simulink model "telemetria_ahrs"  (R2020b)
settings: Solver=FixedStepAuto  StartTime=0.0  StopTime=inf  RelTol=1e-3  EnableMultiTasking=on
libraries: simulink_extras x11, svdutilitieslib x2, arduinolib x1
(part 1 of 2)
settings Model: SILPILModeSetting=veronly  ExtModeTrigDuration=2  Creator=ricca  LastModifiedBy=lapis-dspace
settings SolverCC: AutoInsertRateTranBlk=on
settings OptimizationCC: EnhancedBackFolding=on  PassReuseOutputArgsAs=Individual arguments  ZeroExternalMemoryAtStartup=off  ZeroInternalMemoryAtStartup=off  MaxStackSize=64  OptimizeBlockOrder=speed  DifferentSizesBufferReuse=on  OptimizationCustomize=off  EfficientTunableParamExpr=on
settings DebuggingCC: ParameterTunabilityLossMsg=error
settings HardwareCC: ProdBitPerPointer=32  ProdBitPerSizeT=32  ProdBitPerPtrDiffT=32  ProdLargestAtomicInteger=Long  ProdLargestAtomicFloat=Double  ProdWordSize=32  ProdHWDeviceType=ARM Compatible->ARM Cortex
settings SFSimCC: MATLABDynamicMemAlloc=off
settings RTWCC: Description=Embedded Coder  SystemTargetFile=ert.tlc  HardwareBoard=Arduino Due  TemplateMakefile=ert_default_tmf  Toolchain=Arduino ARM  BuildConfiguration=Faster Runs
settings CodeAppCC: ForceParamTrailComments=on  IgnoreCustomStorageClasses=off  OperatorAnnotations=on  SimulinkDataObjDesc=on  SFDataObjDesc=on  InsertBlockDesc=on
settings ERTTargetCC: SupportContinuousTime=on  SupportVariableSizeSignals=on  ExtModeTransport=3  ExtModeStaticAllocSize=24576  ExtModeMexFile=ext_xcp  ExtModeIntrfLevel=Level2 - Open

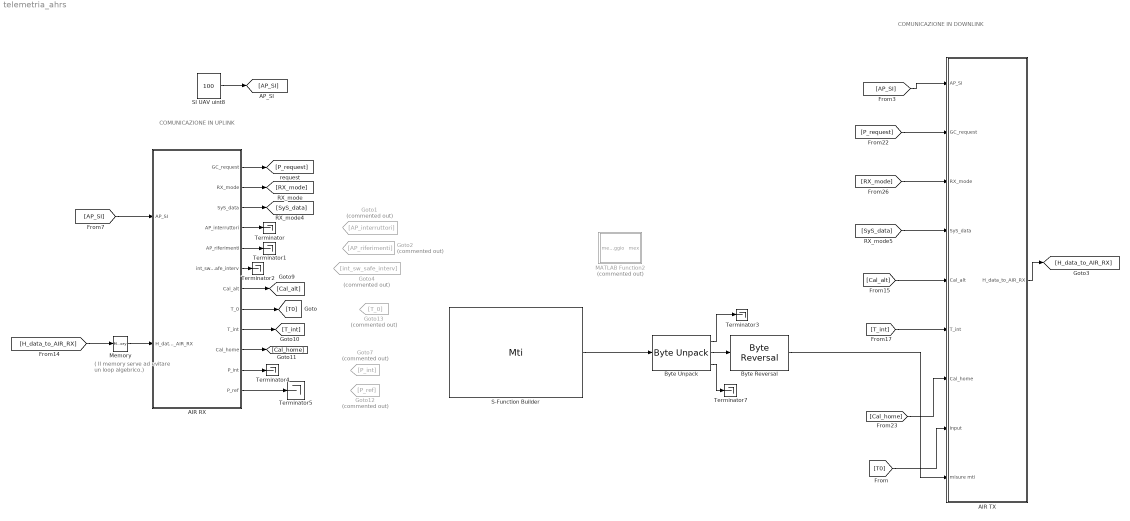
== system telemetria_ahrs ==
  note: ( Il memory serve ad evitare
      | un loop algebrico.)
  note: COMUNICAZIONE IN UPLINK
  note: COMUNICAZIONE IN DOWNLINK
  AIR RX : Subsystem
  AIR TX : Subsystem
  Byte Reversal : svdutilitieslib/Byte Reversal  numInp=1  blockPlatform=arduinoert
      settings: SourceProductBaseCode=ANDROID,ARDUINO,ML_ARDUINO,ECCORTEXA,ECCORTEXR,SC_BEAGLEBONE_BLUE,EC_FREEDOM_BOARD,EC_FRDM_K64F,INTEL_BLOCKSET,JETSONCPU,MICROBIT,NUCLEO,NVIDIA,PX4AUTOPILOTS,RASPPIIO,STMICRODIS,TIC2000,XILINX_BLOCKSET
  Byte Unpack : svdutilitieslib/Byte Unpack  dimensions={[4],[9],[1]}  datatypes={'uint8','single','uint8'}  byteAlign=1  blockPlatform=arduinoert
      settings: SourceProductBaseCode=ANDROID,ARDUINO,ML_ARDUINO,ECCORTEXA,ECCORTEXR,SC_BEAGLEBONE_BLUE,EC_FREEDOM_BOARD,EC_FRDM_K64F,INTEL_BLOCKSET,JETSONCPU,MICROBIT,NUCLEO,NVIDIA,PX4AUTOPILOTS,RASPPIIO,STMICRODIS,TIC2000,XILINX_BLOCKSET
  Goto1 : Goto  Commented=on  GotoTag=AP_interruttori
  Goto12 : Goto  Commented=on  GotoTag=P_ref
  Goto13 : Goto  Commented=on  GotoTag=T_0
  Goto2 : Goto  Commented=on  GotoTag=AP_riferimenti
  Goto4 : Goto  Commented=on  GotoTag=int_sw_safe_interv
  Goto7 : Goto  Commented=on  GotoTag=P_int
  MATLAB Function2 : MATLAB Function  Commented=on  TreatAsAtomicUnit=on
  Memory : Memory
  S-Function Builder : S-Function  InitFcn=try, set_param(gcb,'FunctionName','Mti'), end  FunctionName=Mti  SFunctionModules=Mti_wrapper  SFunctionDeploymentMode=off  EnableBusSupport=off  mask(S-Function Builder){}
      mask help: Simulink:masks:SFunctionBuilder_MD
      mask init:
      | val = [[.9  0.75 0.75 1 1 .9 .9 1]',[1 1 0.75 0.75 .9 .9 1 .9]'];try , sys = get_param(gcb,'SfunBuilderFcnName');if isempty(sys), sys = get_param(gcb,'FunctionName'); end,catch, sys = get_param(gcb,'FunctionName'); end
      settings: CopyFcn=set_param(gcbh,'LinkStatus','none')  PreSaveFcn=try, set_param(gcb,'FunctionName','Mti'), end  OpenFcn=sfunctionwizard(gcbh)
      mask Display: plot(val(:,1),val(:,2)),disp(sys),port_label('output',1,'messaggio')
  SI UAV uint8 : Constant  Value=100  OutDataTypeStr=uint8
  Terminator{,1..5,7} (7 alike) : Terminator
  wires:
  AIR RX/7(Cal_alt) -> [Cal_alt]
  AIR RX/12(P_ref) -> Terminator5/1
  [AP_SI] -> AIR RX/1(AP_SI)
  [H_data_to_AIR_RX] -> Memory/1
  AIR RX/8(T_0) -> [T0]
  AIR RX/10(Cal_home) -> [Cal_home]
  AIR RX/9(T_int) -> [T_int]
  AIR RX/6(int_sw_safe_interv) -> Terminator2/1
  AIR RX/1(GC_request) -> [P_request]
  Memory/1 -> AIR RX/2(H_data_to_AIR_RX)
  AIR RX/2(RX_mode) -> [RX_mode]
  AIR RX/5(AP_riferimenti) -> Terminator1/1
  AIR RX/11(P_int) -> Terminator4/1
  AIR RX/4(AP_interruttori) -> Terminator/1
  AIR RX/3(SyS_data) -> [SyS_data]
  SI UAV uint8/1 -> [AP_SI]
  AIR TX/1(H_data_to_AIR_RX) -> [H_data_to_AIR_RX]
  [AP_SI] -> AIR TX/1(AP_SI)
  [Cal_alt] -> AIR TX/5(Cal_alt)
  [P_request] -> AIR TX/2(GC_request)
  [T_int] -> AIR TX/6(T_int)
  [RX_mode] -> AIR TX/3(RX_mode)
  [SyS_data] -> AIR TX/4(SyS_data)
  [Cal_home] -> AIR TX/7(Cal_home)
  [T0] -> AIR TX/8(Input)
  Byte Unpack/1 -> Terminator3/1
  Byte Unpack/2 -> Byte Reversal/1
  Byte Unpack/3 -> Terminator7/1
  S-Function Builder/1 -> Byte Unpack/1
  Byte Reversal/1 -> AIR TX/9(misure mti)

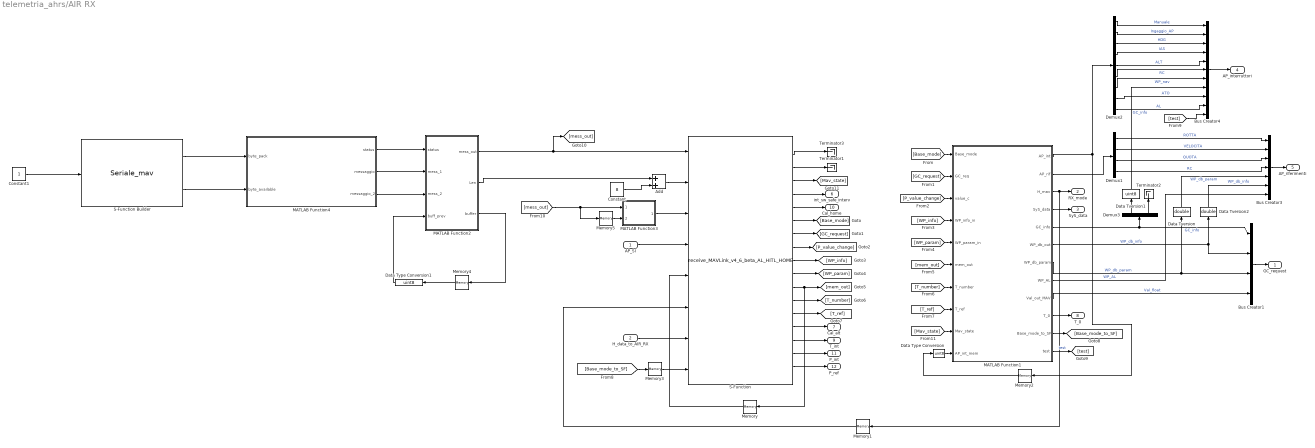
== system telemetria_ahrs/AIR RX ==
  AP_SI : Inport
  H_data_to_AIR_RX : Inport  Port=2
  Add : Sum  AccumDataTypeStr=int32
  Bus Creator1 : BusCreator  Inputs=4
  Bus Creator3 : BusCreator  Inputs=7
  Bus Creator4 : BusCreator  Inputs=11
  Constant : Constant  Value=8  OutDataTypeStr=int32  SampleTime=-1
  Constant1 : Constant  OutDataTypeStr=uint8
  Data Tversion : DataTypeConversion  OutDataTypeStr=double
  Data Tversion1 : DataTypeConversion  OutDataTypeStr=uint8
  Data Tversion2 : DataTypeConversion  OutDataTypeStr=double
  Data Type Conversion : DataTypeConversion  OutDataTypeStr=uint8
  Data Type Conversion1 : DataTypeConversion  OutDataTypeStr=uint8
  Demux1 : Demux
  Demux2 : Demux  Outputs=9
  Demux3 : Demux  Outputs=[1 2]
  MATLAB Function1 : MATLAB Function  TreatAsAtomicUnit=on
  MATLAB Function2 : MATLAB Function  TreatAsAtomicUnit=on
  MATLAB Function3 : MATLAB Function  TreatAsAtomicUnit=on
  MATLAB Function4 : MATLAB Function  TreatAsAtomicUnit=on
  Memory : Memory  InheritSampleTime=on
  Memory1 : Memory  InheritSampleTime=on
  Memory2 : Memory  InitialCondition=[0 0 0 0 0 0 0 0 0]
  Memory3 : Memory
  Memory4 : Memory  InitialCondition=uint8(zeros(3,100))  InheritSampleTime=on
  Memory5 : Memory  InheritSampleTime=on
  S-Function : S-Function  FunctionName=receive_MAVLink_v4_6_beta_AL_HITL_HOME  SFunctionModules='receive_MAVLink_v4_6_beta_AL_HITL_HOME_wrapper'  SFunctionDeploymentMode=off  EnableBusSupport=off
  S-Function Builder : S-Function  InitFcn=try, set_param(gcb,'FunctionName','Seriale_mav'), end  FunctionName=Seriale_mav  SFunctionModules=Seriale_mav_wrapper  SFunctionDeploymentMode=off  EnableBusSupport=off  mask(S-Function Builder){}
      mask help: Simulink:masks:SFunctionBuilder_MD
      mask init: same as telemetria_ahrs/S-Function Builder
      settings: CopyFcn=set_param(gcbh,'LinkStatus','none')  PreSaveFcn=try, set_param(gcb,'FunctionName','Seriale_mav'), end  OpenFcn=sfunctionwizard(gcbh)
      mask Display: plot(val(:,1),val(:,2)),disp(sys),port_label('input',1,'inutile'),port_label('output',1,'Messaggio'),port_label('output',2,'serial_available')
  Terminator1 : Terminator
  Terminator2 : Terminator
  Terminator3 : Terminator
  GC_request : Outport  VectorParamsAs1DForOutWhenUnconnected=off
  RX_mode : Outport  Port=2  VectorParamsAs1DForOutWhenUnconnected=off
  SyS_data : Outport  Port=3  VectorParamsAs1DForOutWhenUnconnected=off
  AP_interruttori : Outport  Port=4  VectorParamsAs1DForOutWhenUnconnected=off
  AP_riferimenti : Outport  Port=5  VectorParamsAs1DForOutWhenUnconnected=off
  int_sw_safe_interv : Outport  Port=6  VectorParamsAs1DForOutWhenUnconnected=off
  Cal_alt : Outport  Port=7  VectorParamsAs1DForOutWhenUnconnected=off
  T_0 : Outport  Port=8  VectorParamsAs1DForOutWhenUnconnected=off
  T_int : Outport  Port=9  VectorParamsAs1DForOutWhenUnconnected=off
  Cal_home : Outport  Port=10  VectorParamsAs1DForOutWhenUnconnected=off
  P_int : Outport  Port=11  VectorParamsAs1DForOutWhenUnconnected=off
  P_ref : Outport  Port=12  VectorParamsAs1DForOutWhenUnconnected=off
  wires:
  H_data_to_AIR_RX/1 -> S-Function/7
  Memory1/1 -> S-Function/6
  Memory/1 -> S-Function/5
  Memory3/1 -> S-Function/8
  AP_SI/1 -> S-Function/4
  S-Function/5 -> Cal_home/1
  S-Function/4 -> int_sw_safe_interv/1
  S-Function/3 -> [Mav_state]
  S-Function/2 -> Terminator1/1
  S-Function/1 -> Terminator3/1
  S-Function/15 -> T_int/1
  S-Function/14 -> Cal_alt/1
  S-Function/13 -> [T_ref]
  S-Function/12 -> [T_number]
  S-Function/11 -> Memory/1, [mem_out]
  S-Function/10 -> [WP_param]
  S-Function/9 -> [WP_info]
  S-Function/8 -> [P_value_change]
  S-Function/6 -> [Base_mode]
  S-Function/7 -> [GC_request]
  Demux2/6 -> Bus Creator4/6  "RC"
  Data Tversion1/1 -> Bus Creator4/8  "GC_info"
  Memory2/1 -> Data Type Conversion/1
  Bus Creator1/1 -> GC_request/1
  Demux1/2 -> Bus Creator3/2  "VELOCITA"
  Demux2/5 -> Bus Creator4/5  "ALT"
  Demux2/1 -> Bus Creator4/1  "Manuale"
  Demux2/3 -> Bus Creator4/3  "HDG"
  [P_value_change] -> MATLAB Function1/3(value_c)
  Demux1/4 -> Bus Creator3/4  "RC"
  MATLAB Function1/2(AP_rif) -> Demux1/1
  Demux2/8 -> Bus Creator4/9  "ATO"
  MATLAB Function1/7(WP_db_param) -> Bus Creator1/3, Data Tversion/1  "WP_db_param"
  [GC_request] -> MATLAB Function1/2(GC_req)
  Demux2/2 -> Bus Creator4/2  "Ingaggio_AP"
  [mem_out] -> MATLAB Function1/6(mem_out)
  Bus Creator4/1 -> AP_interruttori/1
  MATLAB Function1/4(SyS_data) -> SyS_data/1
  MATLAB Function1/6(WP_db_out) -> Data Tversion2/1, Bus Creator1/2  "WP_db_info"
  [Mav_state] -> MATLAB Function1/9(Mav_state)
  Demux2/7 -> Bus Creator4/7  "WP_nav"
  [T_ref] -> MATLAB Function1/8(T_ref)
  Data Type Conversion/1 -> MATLAB Function1/10(AP_int_mem)
  Data Tversion2/1 -> Bus Creator3/6  "WP_db_info"
  Demux3/2 -> Terminator2/1
  [Base_mode] -> MATLAB Function1/1(Base_mode)
  [WP_param] -> MATLAB Function1/5(WP_param_in)
  Data Tversion/1 -> Bus Creator3/5  "WP_db_param"
  Demux3/1 -> Data Tversion1/1
  MATLAB Function1/3(H_mav) -> Memory1/1, RX_mode/1
  MATLAB Function1/9(Val_out_MAV) -> Bus Creator1/4  "Val_float"
  Bus Creator3/1 -> AP_riferimenti/1
  [T_number] -> MATLAB Function1/7(T_number)
  MATLAB Function1/5(GC_info) -> Demux3/1, Bus Creator1/1  "GC_info"
  MATLAB Function1/1(AP_int) -> Demux2/1, Memory2/1
  [WP_info] -> MATLAB Function1/4(WP_info_in)
  [Base_mode_to_SF] -> Memory3/1
  MATLAB Function1/11(Base_mode_to_SF) -> [Base_mode_to_SF]
  Demux1/3 -> Bus Creator3/3  "QUOTA"
  MATLAB Function1/12(test) -> [test]  "test"
  Demux2/4 -> Bus Creator4/4  "IAS"
  [test] -> Bus Creator4/11
  Demux1/1 -> Bus Creator3/1  "ROTTA"
  MATLAB Function1/8(WP_AL) -> Bus Creator3/7  "WP_AL"
  MATLAB Function1/10(T_0) -> T_0/1
  Demux2/9 -> Bus Creator4/10  "AL"
  MATLAB Function4/3(messaggio_2) -> MATLAB Function2/3(mess_2)
  MATLAB Function2/2(Len) -> Add/1
  MATLAB Function4/1(status) -> MATLAB Function2/1(status)
  MATLAB Function4/2(messaggio) -> MATLAB Function2/2(mess_1)
  Memory4/1 -> Data Type Conversion1/1
  MATLAB Function2/3(buffer) -> Memory4/1
  Constant/1 -> Add/2
  MATLAB Function2/1(mess_out) -> S-Function/1, [mess_out]
  MATLAB Function3/1(new_mex) -> S-Function/3
  Add/1 -> S-Function/2
  Data Type Conversion1/1 -> MATLAB Function2/4(buff_prev)
  Memory5/1 -> MATLAB Function3/2(mess_out_prev)
  [mess_out] -> Memory5/1, MATLAB Function3/1(mess_out)
  S-Function Builder/2 -> MATLAB Function4/2(byte_available)
  S-Function Builder/1 -> MATLAB Function4/1(byte_pack)
  Constant1/1 -> S-Function Builder/1
  S-Function/16 -> P_int/1
  S-Function/17 -> P_ref/1

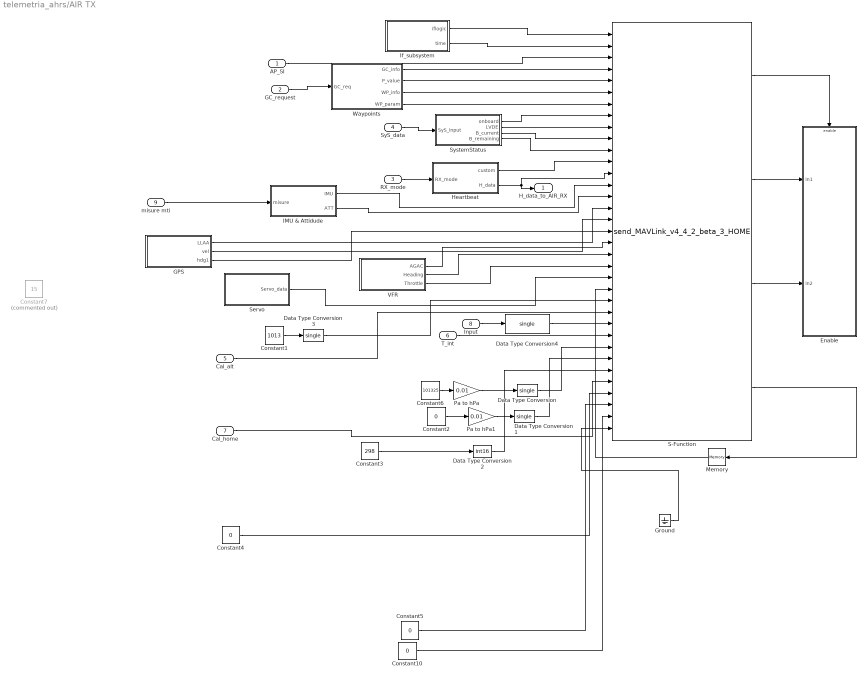
== system telemetria_ahrs/AIR TX ==
  AP_SI : Inport
  GC_request : Inport  Port=2
  RX_mode : Inport  Port=3
  SyS_data : Inport  Port=4
  Cal_alt : Inport  Port=5
  T_int : Inport  Port=6
  Cal_home : Inport  Port=7
  Input : Inport  Port=8
  misure mti : Inport  Port=9
  Constant1 : Constant  Value=1013
  Constant{2,4..5,10} (4 alike) : Constant  Value=0
  Constant3 : Constant  Value=298
  Constant6 : Constant  Value=101325
  Constant7 : Constant  Commented=on  Value=15
  Data Type Conversion{,1,3..4} (4 alike) : DataTypeConversion  OutDataTypeStr=single
  Data Type Conversion2 : DataTypeConversion  OutDataTypeStr=int16
  "Enable " : Subsystem  TreatAsAtomicUnit=on
  GPS : Subsystem  SystemSampleTime=0.02
  Ground : Ground
  Heartbeat : Subsystem  SystemSampleTime=1
  IMU & Attidude : Subsystem  SystemSampleTime=0.04
  If_subsystem : Subsystem
  Memory : Memory
  Pa to hPa : Gain  Gain=0.01
  Pa to hPa1 : Gain  Gain=0.01
  S-Function : S-Function  FunctionName=send_MAVLink_v4_4_2_beta_3_HOME  SFunctionModules='send_MAVLink_v4_4_2_beta_3_HOME_wrapper'  SFunctionDeploymentMode=off  EnableBusSupport=off
  Servo : Subsystem  SystemSampleTime=0.5
  SystemStatus : Subsystem  SystemSampleTime=0.2
  VFR : Subsystem  SystemSampleTime=0.5
  Waypoints : Subsystem  SystemSampleTime=1
  H_data_to_AIR_RX : Outport  VectorParamsAs1DForOutWhenUnconnected=off
  wires:
  If_subsystem/2(time) -> S-Function/2
  If_subsystem/1(iflogic) -> S-Function/1
  VFR/2(Heading) -> S-Function/20
  Heartbeat/2(H_data) -> H_data_to_AIR_RX/1, S-Function/13
  RX_mode/1 -> Heartbeat/1(RX_mode)
  S-Function/1 -> "Enable "/Enable
  Input/1 -> Data Type Conversion4/1
  AP_SI/1 -> S-Function/3
  Constant2/1 -> Pa to hPa1/1
  SyS_data/1 -> SystemStatus/1(SyS_input)
  S-Function/3 -> "Enable "/2(In2)
  SystemStatus/1(onboard) -> S-Function/8
  SystemStatus/4(B_remaining) -> S-Function/11
  T_int/1 -> S-Function/27
  SystemStatus/2(LVDE) -> S-Function/9
  Heartbeat/1(custom) -> S-Function/12
  Cal_alt/1 -> S-Function/25
  GC_request/1 -> Waypoints/1(GC_req)
  S-Function/4 -> Memory/1
  S-Function/2 -> "Enable "/1(In1)
  GPS/3(hdg1) -> S-Function/18
  Waypoints/2(P_value) -> S-Function/5
  IMU & Attidude/2(ATT) -> S-Function/15
  Memory/1 -> S-Function/23
  Data Type Conversion1/1 -> S-Function/29
  Waypoints/1(GC_info) -> S-Function/4
  Servo/1(Servo_data) -> S-Function/22
  GPS/2(vel) -> S-Function/17
  IMU & Attidude/1(IMU) -> S-Function/14
  Constant3/1 -> Data Type Conversion2/1
  Waypoints/3(WP_info) -> S-Function/6
  Pa to hPa1/1 -> Data Type Conversion1/1
  Data Type Conversion3/1 -> S-Function/24
  GPS/1(LLAA) -> S-Function/16
  Data Type Conversion2/1 -> S-Function/30
  Constant10/1 -> S-Function/34
  SystemStatus/3(B_current) -> S-Function/10
  Cal_home/1 -> S-Function/31
  VFR/3(Throttle) -> S-Function/21
  Waypoints/4(WP_param) -> S-Function/7
  Constant4/1 -> S-Function/32
  VFR/1(AGAC) -> S-Function/19
  Constant5/1 -> S-Function/33
  Ground/1 -> S-Function/35
  Constant1/1 -> Data Type Conversion3/1
  Constant6/1 -> Pa to hPa/1
  Data Type Conversion/1 -> S-Function/28
  Pa to hPa/1 -> Data Type Conversion/1
  Data Type Conversion4/1 -> S-Function/26
  misure mti/1 -> IMU & Attidude/1(misure)

== system telemetria_ahrs/AIR TX/Enable  ==
  In1 : Inport
  In2 : Inport  Port=2
  Enable : EnablePort
  Chart : Stateflow chart  TreatAsAtomicUnit=on
  wires:
  In2/1 -> Chart/2(Len)
  In1/1 -> Chart/1(datain)

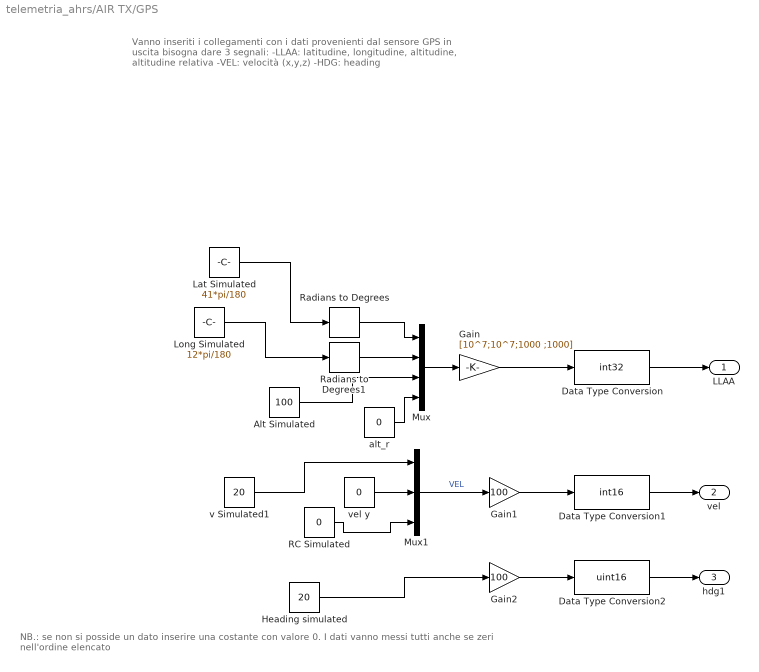
== system telemetria_ahrs/AIR TX/GPS ==
  note: NB.: se non si posside un dato inserire una costante con valore 0. I dati vanno messi tutti anche se zeri nell'ordine elencato
  note: Vanno inseriti i collegamenti con i dati provenienti dal sensore GPS
      | in uscita bisogna dare 3 segnali:
      |
      | -LLAA: latitudine, longitudine, altitudine, altitudine relativa
      | -VEL: velocità (x,y,z)
      | -HDG: heading
  Alt Simulated : Constant  Value=100
  Data Type Conversion : DataTypeConversion  OutDataTypeStr=int32  RndMeth=Simplest
  Data Type Conversion1 : DataTypeConversion  OutDataTypeStr=int16  RndMeth=Simplest
  Data Type Conversion2 : DataTypeConversion  OutDataTypeStr=uint16  RndMeth=Simplest
  Gain : Gain  Gain=[10^7;10^7;1000 ;1000]
  Gain1 : Gain  Gain=100
  Gain2 : Gain  Gain=100
  Heading simulated : Constant  Value=20
  Lat Simulated : Constant  Value=41*pi/180
  Long Simulated : Constant  Value=12*pi/180
  Mux : Mux
  Mux1 : Mux  Inputs=3
  RC Simulated : Constant  Value=0
  Radians to Degrees : simulink_extras/Transformations/Radians to Degrees
  Radians to Degrees1 : simulink_extras/Transformations/Radians to Degrees
  alt_r : Constant  Value=0
  v Simulated1 : Constant  Value=20
  vel y : Constant  Value=0  OutDataTypeStr=double
  LLAA : Outport  VectorParamsAs1DForOutWhenUnconnected=off
  vel : Outport  Port=2  VectorParamsAs1DForOutWhenUnconnected=off
  hdg1 : Outport  Port=3  VectorParamsAs1DForOutWhenUnconnected=off
  wires:
  Lat Simulated/1 -> Radians to Degrees/1
  Long Simulated/1 -> Radians to Degrees1/1
  Alt Simulated/1 -> Mux/3
  Gain2/1 -> Data Type Conversion2/1
  Data Type Conversion/1 -> LLAA/1
  Gain/1 -> Data Type Conversion/1
  Data Type Conversion1/1 -> vel/1
  Radians to Degrees1/1 -> Mux/2
  Radians to Degrees/1 -> Mux/1
  RC Simulated/1 -> Mux1/3
  vel y/1 -> Mux1/2
  Heading simulated/1 -> Gain2/1
  Mux/1 -> Gain/1
  v Simulated1/1 -> Mux1/1
  Mux1/1 -> Gain1/1  "VEL"
  Data Type Conversion2/1 -> hdg1/1
  alt_r/1 -> Mux/4
  Gain1/1 -> Data Type Conversion1/1

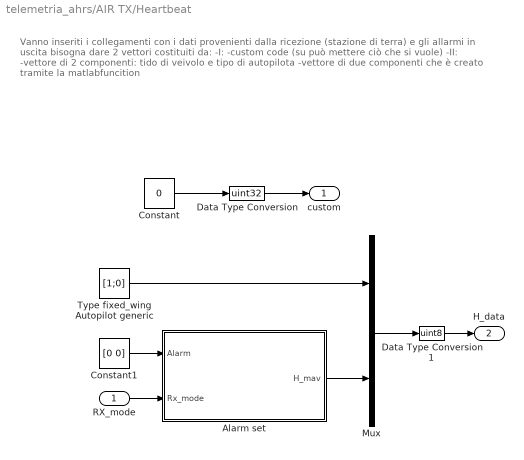
== system telemetria_ahrs/AIR TX/Heartbeat ==
  note: Vanno inseriti i collegamenti con i dati provenienti dalla ricezione (stazione di terra) e gli allarmi
      | in uscita bisogna dare 2 vettori costituiti da:
      | -I:
      | -custom code (su può mettere ciò che si vuole)
      | -II:
      | -vettore di 2 componenti: tido di veivolo e tipo di autopilota
      | -vettore di due componenti che è creato tramite la matlabfuncition
  RX_mode : Inport
  Alarm set : MATLAB Function  TreatAsAtomicUnit=on
  Constant : Constant  Value=0
  Constant1 : Constant  Value=[0 0]
  Data Type Conversion : DataTypeConversion  OutDataTypeStr=uint32
  Data Type Conversion1 : DataTypeConversion  OutDataTypeStr=uint8
  Mux : Mux  Inputs=2
  Type fixed_wing Autopilot generic : Constant  Value=[1;0]  OutDataTypeStr=uint8
  custom : Outport  VectorParamsAs1DForOutWhenUnconnected=off
  H_data : Outport  Port=2  VectorParamsAs1DForOutWhenUnconnected=off
  wires:
  Constant/1 -> Data Type Conversion/1
  Data Type Conversion1/1 -> H_data/1
  Data Type Conversion/1 -> custom/1
  RX_mode/1 -> Alarm set/2(Rx_mode)
  Constant1/1 -> Alarm set/1(Alarm)
  Type fixed_wing Autopilot generic/1 -> Mux/1
  Alarm set/1(H_mav) -> Mux/2
  Mux/1 -> Data Type Conversion1/1

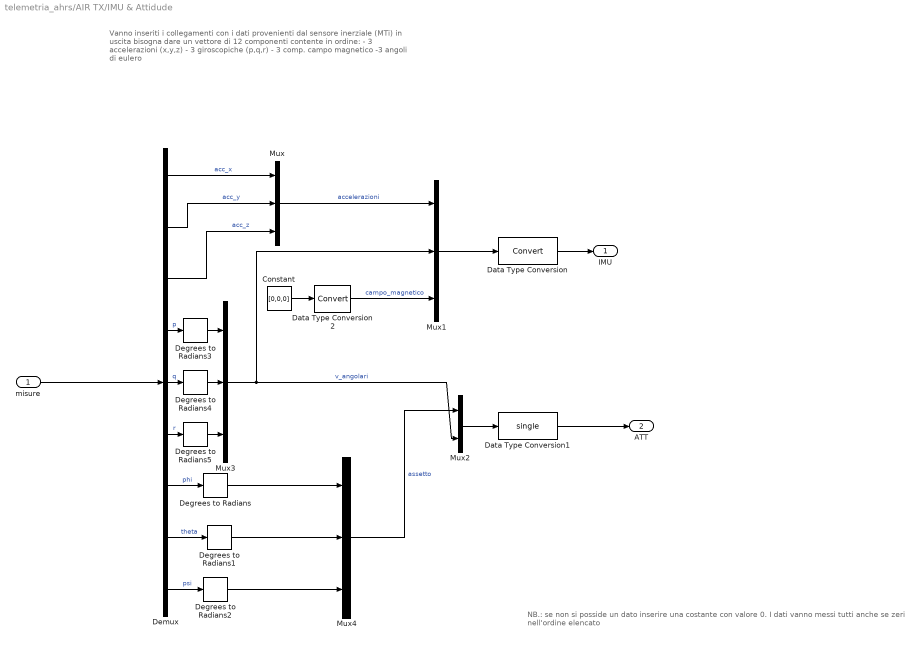
== system telemetria_ahrs/AIR TX/IMU & Attidude ==
  note: Vanno inseriti i collegamenti con i dati provenienti dal sensore inerziale (MTi)
      | in uscita bisogna dare un vettore di 12 componenti contente in ordine:
      | - 3 accelerazioni (x,y,z)
      | - 3 giroscopiche (p,q,r)
      | - 3 comp. campo magnetico
      | -3 angoli di eulero
  note: NB.: se non si posside un dato inserire una costante con valore 0. I dati vanno messi tutti anche se zeri nell'ordine elencato
  misure : Inport
  Constant : Constant  Value=[0,0,0]
  Data Type Conversion : DataTypeConversion
  Data Type Conversion1 : DataTypeConversion  OutDataTypeStr=single
  Data Type Conversion2 : DataTypeConversion
  Degrees to Radians{,1..5} (6 alike) : simulink_extras/Transformations/Degrees to Radians
  Demux : Demux  Outputs=9
  Mux{,1,3..4} (4 alike) : Mux  Inputs=3
  Mux2 : Mux  Inputs=2
  IMU : Outport  VectorParamsAs1DForOutWhenUnconnected=off
  ATT : Outport  Port=2  VectorParamsAs1DForOutWhenUnconnected=off
  wires:
  Demux/4 -> Degrees to Radians3/1  "p"
  Demux/6 -> Degrees to Radians5/1  "r"
  Demux/7 -> Degrees to Radians/1  "phi"
  Demux/9 -> Degrees to Radians2/1  "psi"
  Demux/5 -> Degrees to Radians4/1  "q"
  Demux/8 -> Degrees to Radians1/1  "theta"
  misure/1 -> Demux/1
  Mux/1 -> Mux1/1  "accelerazioni"
  Demux/3 -> Mux/3  "acc_z"
  Mux4/1 -> Mux2/1  "assetto"
  Demux/2 -> Mux/2  "acc_y"
  Mux3/1 -> Mux1/2, Mux2/2  "v_angolari"
  Demux/1 -> Mux/1  "acc_x"
  Mux1/1 -> Data Type Conversion/1
  Mux2/1 -> Data Type Conversion1/1
  Data Type Conversion1/1 -> ATT/1
  Data Type Conversion/1 -> IMU/1
  Constant/1 -> Data Type Conversion2/1
  Data Type Conversion2/1 -> Mux1/3  "campo_magnetico"
  Degrees to Radians2/1 -> Mux4/3
  Degrees to Radians3/1 -> Mux3/1
  Degrees to Radians4/1 -> Mux3/2
  Degrees to Radians5/1 -> Mux3/3
  Degrees to Radians/1 -> Mux4/1
  Degrees to Radians1/1 -> Mux4/2

== system telemetria_ahrs/AIR TX/If_subsystem ==
  note: Blocco per la temporizzazione dell'invio dei messaggi
  Data Type Conversion3 : DataTypeConversion  OutDataTypeStr=uint32  RndMeth=Simplest
  Gain : Gain  Gain=100
  Subsystem : Subsystem
  iflogic_function : MATLAB Function  TreatAsAtomicUnit=on
  iflogic : Outport  VectorParamsAs1DForOutWhenUnconnected=off
  time : Outport  Port=2  VectorParamsAs1DForOutWhenUnconnected=off
  wires:
  Subsystem/3(time) -> Gain/1
  Subsystem/2(H_10) -> iflogic_function/2(H10)
  Subsystem/1(H_50) -> iflogic_function/1(H50)
  Gain/1 -> Data Type Conversion3/1
  Data Type Conversion3/1 -> time/1
  iflogic_function/1(iflogic) -> iflogic/1

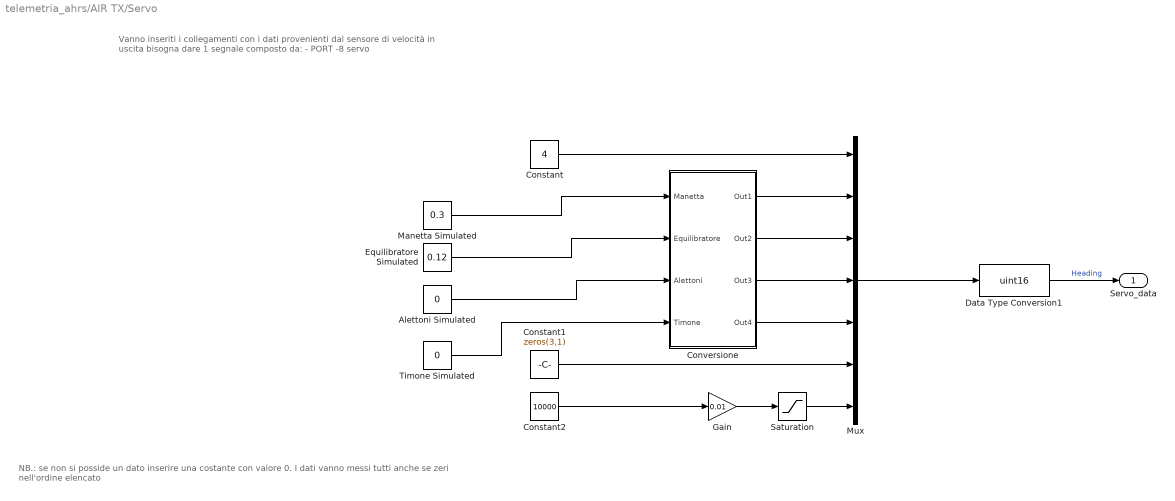
== system telemetria_ahrs/AIR TX/Servo ==
  note: NB.: se non si posside un dato inserire una costante con valore 0. I dati vanno messi tutti anche se zeri nell'ordine elencato
  note: Vanno inseriti i collegamenti con i dati provenienti dal sensore di velocità
      | in uscita bisogna dare 1 segnale composto da:
      |
      | -  PORT
      | -8 servo
  Alettoni Simulated : Constant  Value=0
  Constant : Constant  Value=4
  Constant1 : Constant  Value=zeros(3,1)
  Constant2 : Constant  Value=10000
  Conversione : Subsystem
  Data Type Conversion1 : DataTypeConversion  OutDataTypeStr=uint16  RndMeth=Simplest
  Equilibratore Simulated : Constant  Value=0.12
  Gain : Gain  Gain=0.01
  Manetta Simulated : Constant  Value=0.3
  Mux : Mux  Inputs=7
  Saturation : Saturate  UpperLimit=4000  LowerLimit=0
  Timone Simulated : Constant  Value=0
  Servo_data : Outport  VectorParamsAs1DForOutWhenUnconnected=off
  wires:
  Constant2/1 -> Gain/1
  Equilibratore Simulated/1 -> Conversione/2(Equilibratore)
  Alettoni Simulated/1 -> Conversione/3(Alettoni)
  Timone Simulated/1 -> Conversione/4(Timone)
  Manetta Simulated/1 -> Conversione/1(Manetta)
  Conversione/3(Out3) -> Mux/4
  Constant1/1 -> Mux/6
  Conversione/1(Out1) -> Mux/2
  Mux/1 -> Data Type Conversion1/1
  Constant/1 -> Mux/1
  Data Type Conversion1/1 -> Servo_data/1  "Heading"
  Conversione/4(Out4) -> Mux/5
  Saturation/1 -> Mux/7
  Gain/1 -> Saturation/1
  Conversione/2(Out2) -> Mux/3

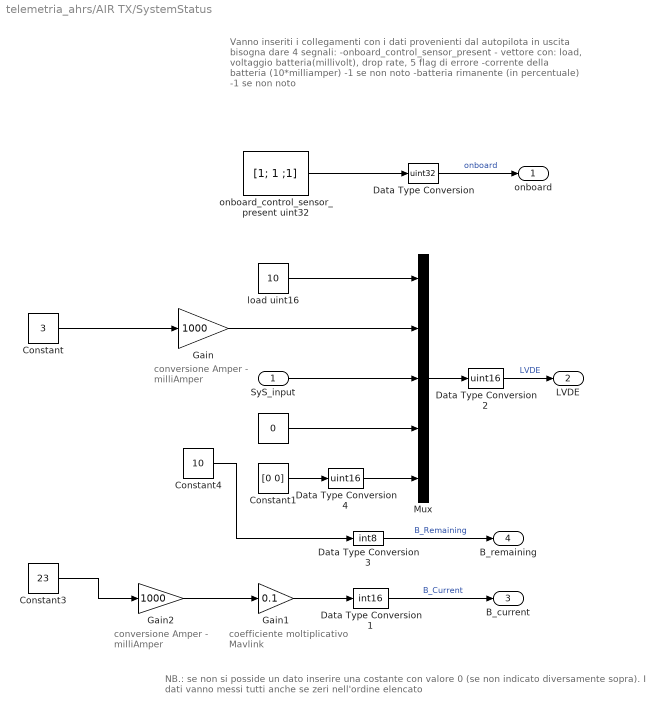
== system telemetria_ahrs/AIR TX/SystemStatus ==
  note: coefficiente moltiplicativo Mavlink
  note: conversione
      | Amper - milliAmper
  note: NB.: se non si posside un dato inserire una costante con valore 0 (se non indicato diversamente sopra).
      | I dati vanno messi tutti anche se zeri nell'ordine elencato
  note: Vanno inseriti i collegamenti con i dati provenienti dal autopilota
      | in uscita bisogna dare 4 segnali:
      |
      | -onboard_control_sensor_present
      | - vettore con: load, voltaggio batteria(millivolt), drop rate, 5 flag di errore
      | -corrente della batteria (10*milliamper) -1 se non noto
      | -batteria rimanente (in percentuale) -1 se non noto
  note: conversione
      | Amper - milliAmper
  SyS_input : Inport
  " " : Constant  Value=0  OutDataTypeStr=uint16
  Constant : Constant  Value=3
  Constant1 : Constant  Value=[0 0]
  Constant3 : Constant  Value=23
  Constant4 : Constant  Value=10
  Data Type Conversion : DataTypeConversion  OutDataTypeStr=uint32
  Data Type Conversion1 : DataTypeConversion  OutDataTypeStr=int16
  Data Type Conversion2 : DataTypeConversion  OutDataTypeStr=uint16
  Data Type Conversion3 : DataTypeConversion  OutDataTypeStr=int8
  Data Type Conversion4 : DataTypeConversion  OutDataTypeStr=uint16
  Gain : Gain  Gain=1000  OutDataTypeStr=uint16
  Gain1 : Gain  Gain=0.1  OutDataTypeStr=int16
  Gain2 : Gain  Gain=1000  OutDataTypeStr=int16
  Mux : Mux  Inputs=5
  load uint16 : Constant  Value=10  OutDataTypeStr=uint16
  onboard_control_sensor_present uint32 : Constant  Value=[1; 1 ;1]  OutDataTypeStr=uint32
  onboard : Outport  VectorParamsAs1DForOutWhenUnconnected=off
  LVDE : Outport  Port=2  VectorParamsAs1DForOutWhenUnconnected=off
  B_current : Outport  Port=3  VectorParamsAs1DForOutWhenUnconnected=off
  B_remaining : Outport  Port=4  VectorParamsAs1DForOutWhenUnconnected=off
  wires:
  Gain2/1 -> Gain1/1
  Gain1/1 -> Data Type Conversion1/1
  " "/1 -> Mux/4
  Data Type Conversion4/1 -> Mux/5
  Constant1/1 -> Data Type Conversion4/1
  SyS_input/1 -> Mux/3
  Data Type Conversion3/1 -> B_remaining/1  "B_Remaining"
  Data Type Conversion1/1 -> B_current/1  "B_Current"
  Data Type Conversion2/1 -> LVDE/1  "LVDE"
  Data Type Conversion/1 -> onboard/1  "onboard"
  Mux/1 -> Data Type Conversion2/1
  Gain/1 -> Mux/2
  load uint16/1 -> Mux/1
  onboard_control_sensor_present uint32/1 -> Data Type Conversion/1
  Constant/1 -> Gain/1
  Constant4/1 -> Data Type Conversion3/1
  Constant3/1 -> Gain2/1

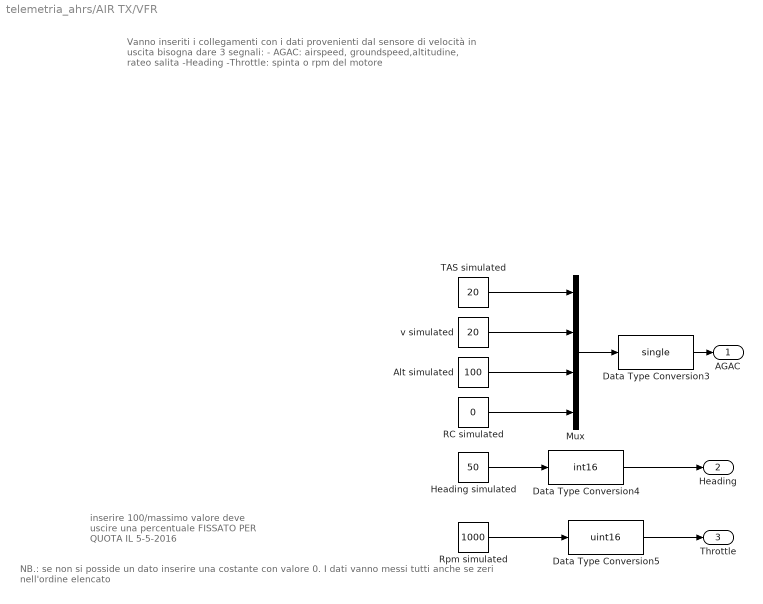
== system telemetria_ahrs/AIR TX/VFR ==
  note: NB.: se non si posside un dato inserire una costante con valore 0. I dati vanno messi tutti anche se zeri nell'ordine elencato
  note: Vanno inseriti i collegamenti con i dati provenienti dal sensore di velocità
      | in uscita bisogna dare 3 segnali:
      |
      | -  AGAC: airspeed, groundspeed,altitudine, rateo salita
      | -Heading
      | -Throttle: spinta o rpm del motore
  note: inserire 100/massimo valore
      | deve uscire una percentuale
      | FISSATO PER QUOTA IL 5-5-2016
  " Heading simulated" : Constant  Value=50
  Alt simulated : Constant  Value=100
  Data Type Conversion3 : DataTypeConversion  OutDataTypeStr=single
  Data Type Conversion4 : DataTypeConversion  OutDataTypeStr=int16
  Data Type Conversion5 : DataTypeConversion  OutDataTypeStr=uint16
  Mux : Mux
  RC simulated : Constant  Value=0
  Rpm simulated : Constant  Value=1000
  TAS simulated : Constant  Value=20
  v simulated : Constant  Value=20
  AGAC : Outport
  Heading : Outport  Port=2
  Throttle : Outport  Port=3
  wires:
  TAS simulated/1 -> Mux/1
  RC simulated/1 -> Mux/4
  Data Type Conversion5/1 -> Throttle/1
  Data Type Conversion4/1 -> Heading/1
  " Heading simulated"/1 -> Data Type Conversion4/1
  Alt simulated/1 -> Mux/3
  Mux/1 -> Data Type Conversion3/1
  Data Type Conversion3/1 -> AGAC/1
  v simulated/1 -> Mux/2
  Rpm simulated/1 -> Data Type Conversion5/1

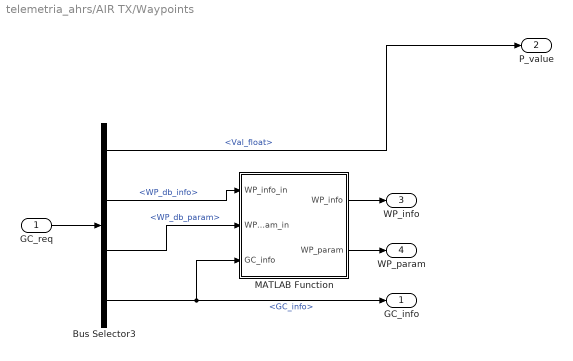
== system telemetria_ahrs/AIR TX/Waypoints ==
  GC_req : Inport
  Bus Selector3 : BusSelector  OutputSignals=Val_float,WP_db_info,WP_db_param,GC_info
  MATLAB Function : MATLAB Function  TreatAsAtomicUnit=on
  GC_info : Outport  VectorParamsAs1DForOutWhenUnconnected=off
  P_value : Outport  Port=2  VectorParamsAs1DForOutWhenUnconnected=off
  WP_info : Outport  Port=3  VectorParamsAs1DForOutWhenUnconnected=off
  WP_param : Outport  Port=4  VectorParamsAs1DForOutWhenUnconnected=off
  wires:
  Bus Selector3/1 -> P_value/1  "<Val_float>"
  MATLAB Function/2(WP_param) -> WP_param/1
  Bus Selector3/3 -> MATLAB Function/2(WP_param_in)  "<WP_db_param>"
  MATLAB Function/1(WP_info) -> WP_info/1
  Bus Selector3/2 -> MATLAB Function/1(WP_info_in)  "<WP_db_info>"
  Bus Selector3/4 -> MATLAB Function/3(GC_info), GC_info/1  "<GC_info>"
  GC_req/1 -> Bus Selector3/1

== system telemetria_ahrs/AIR TX/Enable /Chart/sendbyte ==
  note: sostituito con lo stesso blocco della V. R2015a il 29/1/2016
  bt : Inport  OutDataTypeStr=uint8
  n : Inport  Port=2
  f : TriggerPort  TriggerType=function-call  VariantControl=(inherit)
      settings: CopyFcn=Stateflow.SLINSF.SimulinkMan.removeBlockPreDeleteFcn  PreDeleteFcn=Stateflow.SLINSF.SimulinkMan.unsafePredeleteFcn
  Selector : Selector  InputPortWidth=264  IndexOptions=Index vector (port)  Indices=[1 3]  OutputSizes=1
  Serial Transmit : arduinolib/Serial Transmit  portNumber=2  sendmode=write  sendformat=Decimal  floatprecision=2  blockPlatform=arduino
  wires:
  Selector/1 -> Serial Transmit/1
  n/1 -> Selector/2
  bt/1 -> Selector/1

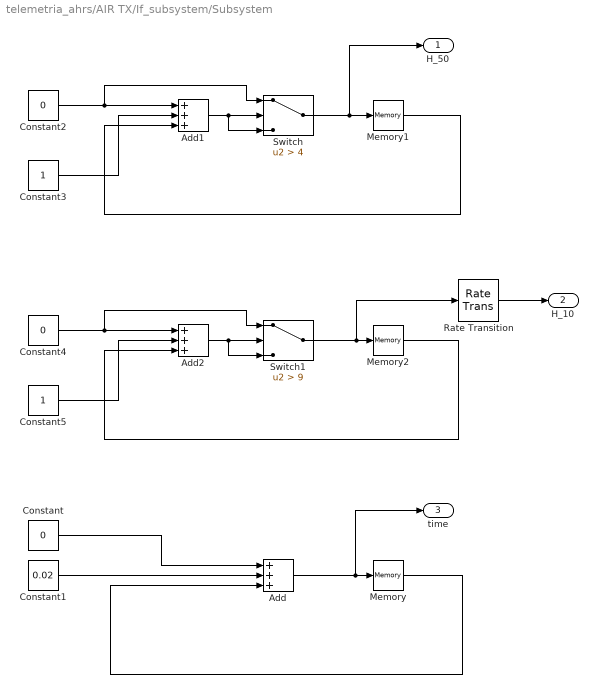
== system telemetria_ahrs/AIR TX/If_subsystem/Subsystem ==
  Add : Sum  Inputs=+++
  Add1 : Sum  Inputs=+++
  Add2 : Sum  Inputs=+++
  Constant : Constant  Value=0  SampleTime=0.02
  Constant1 : Constant  Value=0.02  SampleTime=0.02
  Constant2 : Constant  Value=0  SampleTime=0.02
  Constant3 : Constant  SampleTime=0.02
  Constant4 : Constant  Value=0  SampleTime=0.02*5
  Constant5 : Constant  SampleTime=0.02*5
  Memory : Memory  InitialCondition=-0.02  InheritSampleTime=on
  Memory1 : Memory  InitialCondition=-1  InheritSampleTime=on
  Memory2 : Memory  InitialCondition=-1  InheritSampleTime=on
  Rate Transition : RateTransition  Deterministic=off  OutPortSampleTime=0.02
  Switch : Switch  Criteria=u2 > Threshold  Threshold=4
  Switch1 : Switch  Criteria=u2 > Threshold  Threshold=9
  H_50 : Outport  VectorParamsAs1DForOutWhenUnconnected=off
  H_10 : Outport  Port=2  VectorParamsAs1DForOutWhenUnconnected=off
  time : Outport  Port=3  VectorParamsAs1DForOutWhenUnconnected=off
  wires:
  Memory1/1 -> Add1/3
  Add2/1 -> Switch1/2, Switch1/3
  Constant4/1 -> Add2/1, Switch1/1
  Constant5/1 -> Add2/2
  Memory2/1 -> Add2/3
  Memory/1 -> Add/3
  Add/1 -> time/1, Memory/1
  Constant/1 -> Add/1
  Constant1/1 -> Add/2
  Constant2/1 -> Add1/1, Switch/1
  Switch/1 -> H_50/1, Memory1/1
  Constant3/1 -> Add1/2
  Add1/1 -> Switch/2, Switch/3
  Switch1/1 -> Rate Transition/1, Memory2/1
  Rate Transition/1 -> H_10/1

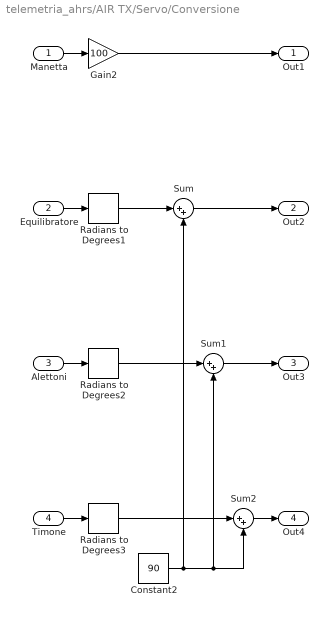
== system telemetria_ahrs/AIR TX/Servo/Conversione ==
  Manetta : Inport
  Equilibratore : Inport  Port=2
  Alettoni : Inport  Port=3
  Timone : Inport  Port=4
  Constant2 : Constant  Value=90
  Gain2 : Gain  Gain=100
  Radians to Degrees1 : simulink_extras/Transformations/Radians to Degrees
  Radians to Degrees2 : simulink_extras/Transformations/Radians to Degrees
  Radians to Degrees3 : simulink_extras/Transformations/Radians to Degrees
  Sum : Sum  Inputs=|++
  Sum1 : Sum  Inputs=|++
  Sum2 : Sum  Inputs=|++
  Out1 : Outport  VectorParamsAs1DForOutWhenUnconnected=off
  Out2 : Outport  Port=2  VectorParamsAs1DForOutWhenUnconnected=off
  Out3 : Outport  Port=3  VectorParamsAs1DForOutWhenUnconnected=off
  Out4 : Outport  Port=4  VectorParamsAs1DForOutWhenUnconnected=off
  wires:
  Sum2/1 -> Out4/1
  Timone/1 -> Radians to Degrees3/1
  Sum1/1 -> Out3/1
  Alettoni/1 -> Radians to Degrees2/1
  Sum/1 -> Out2/1
  Equilibratore/1 -> Radians to Degrees1/1
  Gain2/1 -> Out1/1
  Manetta/1 -> Gain2/1
  Constant2/1 -> Sum2/2, Sum1/2, Sum/2
  Radians to Degrees3/1 -> Sum2/1
  Radians to Degrees2/1 -> Sum1/1
  Radians to Degrees1/1 -> Sum/1

== matlab function telemetria_ahrs/MATLAB Function2 ==
  data: messaggio input; mex output
function mex = fcn(messaggio)
persistent header inviando
if isempty(header)
    header = [250,255,50];
end
if isempty(inviando)
    inviando=[0xFA, 0xFF, 0x32, 0x24, 0xBE, 0xAB, 0xE3, 0x71, 0xBD, 0xE9, 0xD2, 0xC0, 0x41, 0x1D, 0x11, 0x0D, 0xB9, 0xD6, 0x91, 0xF0, 0xBC, 0x01, 0x90, 0x57, 0xBB, 0x07, 0xA3, 0x35, 0xBF, 0x12, 0x4C, 0x38, 0x3F, 0xF5, 0x11, 0x85, 0xC2, 0xE5, 0x3D, 0x09, 0xE0];
    messahex=hex2dec(inviando);
end
if (messaggio(1)==header(1) && messaggio(2)==header(2) && messaggio(3)==header(3))
    mex=messaggio;
else
    mex=messahex;
end

== stateflow chart telemetria_ahrs/AIR TX/Enable /Chart ==
  state sendbyte(bt,n) [function]
  state Inputblock
    entry: i=1;
    Inputblock -> (junction 28)
    (junction 32) -> (junction 28) [order 1] : [ i<Len]
        | {i++;}
    (junction 28) -> (junction 32) : {sendbyte(datain,i);}
    (junction 32) -> (junction 48) [order 2] : {i=1;}
  (default) -> Inputblock
  data: bt function_input uint8; n function_input; datain input uint8; Len input uint16 size=1; i local uint8 =0

== matlab function telemetria_ahrs/AIR TX/Heartbeat/Alarm set ==
  data: Alarm input; H_mav output; Rx_mode input

%%

function H_mav = Allarm_set(Alarm, Rx_mode)
%#cambia lo stato se c'è un allarme attivo
% Allarm: possibili allarmi proveniente dall'autopilota
% Rx_mode: richiesta da parte della stazione di terra
% H_mav: setto i parametri Base_mode e System_status del Heartbeat


H_mav = uint8(Rx_mode); % setta la modalità con quella ricevuta da terra

% se un allarme si attiva ha la precedenza sulla richiesta della QGC

if Alarm(1) == 1 % ovvero l'aereo è entrato in safe e si pone su traettoria circolare di sicurezza
    
    H_mav(1) = uint8(220); % MAV_MODE_AUTO_ARMED
    H_mav(2) = uint8(5);   % MAV_STATE_CRITICAL
%     H_mav(3) = uint8(128); % MAV_MODE_FLAG_SAFETY_ARMED

end

% se l'allareme di intervento pilota è attivo ha precedenza sull'allarm
% sefe per cui bisogna riscrivere lo stato del pilota

if Alarm(2) == 1 % si è attivato l'allarme dell'intervento pilota 
    
    H_mav(1) = uint8(216); % MAV_MODE_GUIDED_ARMED
    H_mav(2) = uint8(4);   % MAV_STATE_ACTIVE
%     H_mav(3) = uint8(8);   % MAV_MODE_FLAG_GUIDED_ENABLED

end

== matlab function telemetria_ahrs/AIR TX/If_subsystem/iflogic_function ==
  data: H50 input; iflogic output; H10 input
function iflogic = fcn(H50,H10)
%#codegen
% prende in ingeresso i counter che contano il tempo
% e dice quale messaggio bisogna inviare in base alle frequenze scelte in
% Heartbeat:            1Hz
% SCALED_IMU:           20Hz
%attitude:              20Hz
%GLOBAL_POSITION_INT:   1Hz
%SYS_STATUS:            3Hz
%VFR_HUD:               2Hz
%SERVO_OUTPUT_RAW       1Hz
%SCALED_PRESSURE        1Hz

if H50 == 1  || H50==3
    iflogic=uint8(26); % SCALED_IMU 20Hz
elseif H50==2 || H50==4
    iflogic=uint8(30); %attitude 20Hz
elseif  H50==0 && H10==2
    iflogic=uint8(33); %GLOBAL_POSITION_INT 1Hz
elseif  H50==0 && H10==6
    iflogic=uint8(34); %GLOBAL_POSITION_INT_RAW 1Hz
elseif  H50==0 && H10==0
    iflogic=uint8(0); %Heartbeat 1Hz
elseif H50==0 && (H10==1 || H10==5 || H10==9)
    iflogic=uint8(1); %SYS_STATUS 3Hz
elseif H50==0 && (H10==3 || H10==8)
    iflogic=uint8(74); %VFR_HUD 2Hz
elseif H50==0 && (H10==7)
    iflogic=uint8(36); %SERVO_OUTPUT_RAW 1Hz
elseif H50==0 && (H10==4)
    iflogic=uint8(29); %SCALED_PRESSURE 1Hz
else
    iflogic=uint8(255); %non esiste nessun messaggio con questo codice
    
end

== matlab function telemetria_ahrs/AIR TX/Waypoints/MATLAB Function ==
  data: WP_info_in input; WP_param_in input; WP_info output; GC_info input; WP_param output
function [WP_info,WP_param] = fcn(WP_info_in,WP_param_in, GC_info)
%#codegen
WP_info=WP_info_in(1,:); %%per sicurezza
WP_param=WP_param_in(1,:); %%per sicurezza
[m,n]=size(WP_info_in);
if GC_info(1)==2
    if GC_info(2)>=0 && GC_info(2)<m %per poter inviare i MISSION_ITEM
        WP_info=WP_info_in(GC_info(2)+1,:);
        WP_param=WP_param_in(GC_info(2)+1,:);
    end
end
if GC_info(1)==3 && GC_info(2)>=0 && GC_info(2)<200 %per poter inviae i MISSION_REQUEST
    WP_info=WP_info_in(GC_info(2)+1,:);
end

== matlab function telemetria_ahrs/AIR RX/MATLAB Function1 ==
  data: Base_mode input; GC_req input; value_c input; WP_info_in input; WP_param_in input; mem_out input; T_number input; T_ref input; Mav_state input; AP_int output; AP_rif output; H_mav output; SyS_data output; GC_info output; WP_db_out output; WP_db_param output; WP_AL output; Val_out_MAV output; T_0 output; AP_int_mem input; Base_mode_to_SF output; test output
function [AP_int, AP_rif, H_mav, SyS_data, GC_info, WP_db_out, WP_db_param,WP_AL, Val_out_MAV, T_0, Base_mode_to_SF, test] =...
    RXelaborazione(Base_mode, GC_req, value_c, WP_info_in, WP_param_in, mem_out, T_number, T_ref, Mav_state, AP_int_mem)
%#codegen
% PARTE PER LA GESTIONE DELLE RICHIESTE DALLA STAZIONE DI TERRA
% GC_req= richiesta della stazione di terra, vettore 2 componenti
%           GC_req(1)=1 :    inviare i parametri a fronte della ricezione del
%                           SET_Request
%                             se GC_req(2)=255 li invia tutti altrimenti
%                             solo 1
% value_c= valore da aggiornare;
% GC_info= necessario per S-function mavlink di trasmissione dipende dal
%               GC_req ricevuto
% WP_db_info= [WP_item255.count,WP_item255.seq,WP_item255.command,WP_item255.frame,
%               WP_item255.current,WP_info[5]=WP_item255.autocontinue]
% WP_db_param= parametri ultimo wp arrivato
% Val_out_MAV= valori aggiornati in uscita per il mavlink di trasmissione
% 
%  mem_out=[msg.sysid; msg.compid;msg.msgid;msg.len;msg.seq;flag]
%
% PARTE PER LA GESTIONE MANUALE AUTOMATICO
%Base_mode: richiesta da parte della stazione di terra di settare una
%           modalità di volo
%H_mav: setto i parametri Base_mode e System_status del Heartbeat di
%           trasmissione
%
%  VARIABILI NECESSARIE ALL'AUTOPILOTA
%AP_interruttori: interruttore di pilota automatico e manuale e modalità
%            [ manuale automatico HDG IAS ALT RC]
%
%AP_riferimenti: valori delle modalità di volo [HDG IAS ALT RC]

persistent riferimenti   % riferimenti delle modalità di volo
persistent WP_dbP WP_dbI WP_dbP_AL % lista dei parametri dei waypoint
persistent test1

nWPmax = uint16(6); % Numero massimo di WP da memorizzare %[MILONE]

% Inizializzazione

if isempty(riferimenti)
    
    riferimenti = single([0; 0; 0; 0; 0; 0; 0; 0; 20; 100; 2; 101325; 15; 0; 0; 0]) ; %valori di riferimento di ["I_HDG", "I_IAS", "I_ALT", "I_RC", "I_WP", "I_ATO", "I_AL" "V_HDG","V_IAS","V_ALT","V_RC","C_P0","C_T0","H_LAT","H_LONG","H_ALT"};]
    
end

if isempty(WP_dbP) || (GC_req(1) == 3 && GC_req(2) == 250)
    
        WP_dbP = single(zeros(nWPmax,7)); % nWPmax righe e 7 colonne
        WP_dbI = uint16(zeros(nWPmax,6)); % nWPmax righe e 6 colonne
        
        
end
if isempty(WP_dbP_AL) || (GC_req(1) == 3 && GC_req(2) == 250)                % introdotto da Sensolini: consente di inviare contemporaneamente wp di navigazione ed atterraggio
    
        WP_dbP_AL = single(zeros(nWPmax,7)); % nWPmax righe e 7 colonne
              
end

if isempty(test1)
    
    test1 = 0;
    
end


%% Parte di richieste da mavlik relativa al messaggio PARAM_SET

GC_info = [GC_req; mem_out(1)]; % GC_req (vettore di due) sarebbe GC_request nella S-Function ed è usato per la funzione di PARAM_SET; 
                                % mem_out(1) sarebbe nella S-Function mem_out[0]=msg.sysid; cioè chi interroga

if GC_info(1) == 1
    
    if GC_info(2) > 0 && GC_info(2) <= 7
        
        if abs(value_c) > 0 % attiva l'interruttore
            
            riferimenti(GC_info(2)) = single(1);
            
            %NB: se arrivano valori maggiori di 1 sempre 1 da in output perchè
            % gli interruttori possono essere solo di tipo 0/1
            % altrimenti l'autopilota si blocca
            
        elseif value_c == 0 % disattiva l'interruttore
            
            riferimenti(GC_info(2)) = single(0);
            
        end
        
    elseif GC_info(2) > 7 && GC_info(2) < 12
        
        riferimenti(GC_info(2)) = single(value_c);
        
    end
    
end

%% Parte relativa al messaggio COMMAND_LONG per la temperatura di riferimento dell'altimetro

if T_number == 13;
    
        riferimenti(T_number) = T_ref;
        
end

%%

Val_out_MAV = riferimenti; % output riferimenti

%% WP set

if GC_info(1) == 3 && GC_info(2) == 200 % arriva il numero dei waypoint
    
     if WP_info_in(1) > nWPmax  %%%ATTENZIONE!!  %[MILONE]
        WP_info_in(1) = nWPmax; % se nWP>nWPmax mi comporto come se avessi ricevuto solo i primi nWPmax
                                % non è ottimale, infatti QGC deve aspettare il time out, ma funziona
                                % va migliorata con una opportuna segnalazione
     end
     
     WP_dbI(:,1) = WP_info_in(1);
     
end

if GC_info(1) == 3 && GC_info(2) < 200 % è arrivato un waypoint
    
    if WP_param_in(2) == 0
    
    WP_dbP(WP_info_in(2)+1,:)   = single(WP_param_in); % 7Parametri. è arrivato il numero WP_info(2) +1 perchè in C si parte da 0
    WP_dbI(WP_info_in(2)+1,2:7) = WP_info_in(2:7);     % 6informazioni. è arrivato il numero WP_info(2)  +1 perchè in C si parte da 0
    
    else
     WP_dbP_AL(WP_param_in(1)+1,:) = single(WP_param_in);
     WP_dbI(WP_info_in(2)+1,2:7) = WP_info_in(2:7);
     
    end
    
end

WP_db_out   = WP_dbI;

WP_db_param = WP_dbP;
WP_AL = WP_dbP_AL;

%for i=1:WP_info_in(1)
%if WP_dbP(WP_info_in(2)+1,2) == 0
%    WP_db_param = WP_dbP;
%    WP_AL = single(zeros(nWPmax,7));
%else
%    WP_db_param = single(zeros(nWPmax,7));
%    WP_AL = WP_dbP;
%end
%end
%% parte di gestione modalità autopilota

H_mav   = uint8(zeros(2,1)); % inizializzo il vettore di output
AP_mode = uint8([0;0]);      % inizializzo il vettore che gli interrutori manuale e automatico

Base_mode_to_SF = uint8(0);

% setto i parametri necessari per l'hearbeat e per l'autopilota

if Base_mode == uint8(0) && Mav_state == uint8(0) % INIZIO: è la condizione che si verifica quando connetto Arduino a QGC, ovvero l'autopilota è in stato Standby
    
    H_mav(1) = uint8(0);         % MAV_MODE_PREFLIGHT
    H_mav(2) = uint8(3);         % MAV_STATE_STANDBY
%     H_mav(3) = uint8(64);        % MAV_MODE_FLAG_MANUAL_INPUT_ENABLED   %% il MAV_MODE_FLAG è commentato perché non lo utilizziamo dato che inviamo nel messaggio dell'heartbeat il MAV_MODE in corrispondenza del valore di base_mode (vedere la pagina web MAV'RIC)
    AP_mode  = uint8([1; 0]);    % attivo il manuale  spengo l'automatico
    Base_mode_to_SF = uint8(0);

elseif Base_mode == uint8(0) && Mav_state == uint8(3) % è arrivato MAV_MODE_PREFLIGHT e MAV_STATE_STANDBY (modalità Ready)
    
    H_mav(1) = uint8(0);         % MAV_MODE_PREFLIGHT
    H_mav(2) = uint8(3);         % MAV_STATE_STANDBY
%     H_mav(3) = uint8(64);        % MAV_MODE_FLAG_MANUAL_INPUT_ENABLED 
    AP_mode  = uint8([1; 0]);    % attivo il manuale  spengo l'automatico
    Base_mode_to_SF = uint8(0);
    test1 = 0;

elseif Base_mode == uint8(0) && Mav_state == uint8(2) % è arrivato MAV_MODE_PREFLIGHT e MAV_STATE_CALIBRATING
    
    H_mav(1) = uint8(0);         % MAV_MODE_PREFLIGHT
    H_mav(2) = uint8(2);         % MAV_STATE_CALIBRATING
%     H_mav(3) = uint8(64);        % MAV_MODE_FLAG_MANUAL_INPUT_ENABLED
    AP_mode  = uint8([1; 0]);    % attivo il manuale  spengo l'automatico
    Base_mode_to_SF = uint8(0);
    test1 = 0;
    
elseif Base_mode == uint8(0) && Mav_state == uint8(1) % è arrivato MAV_MODE_PREFLIGHT e MAV_STATE_BOOT
    
    H_mav(1) = uint8(0);         % MAV_MODE_PREFLIGHT
    H_mav(2) = uint8(1);         % MAV_STATE_BOOT
%     H_mav(3) = uint8(64);        % MAV_MODE_FLAG_MANUAL_INPUT_ENABLED
    AP_mode  = uint8([0; 1]);    % In questo caso si attiva l'interrutore di modalità automatica. 
                                 % Il motivo è dovuto al fatto che per fare la prova del safe è necessario che sia attivo 
                                 % il modo automatico altrimenti il safe non entra.
    Base_mode_to_SF = uint8(0);
    test1 = 1;
    
% elseif Base_mode==uint8(80)  %è arrivato MAV_MODE_STABILIZE_DISARMED, 1 manual in QGC
%     H_mav(1)=uint8(80);        %MAV_MODE_GUIDED_ARMED
%     H_mav(2)=uint8(4);          %MAV_STATE_ACTIVE
%     AP_mode=uint8([1; 0]);      %attivo il manuale  spengo l'automatico

elseif Base_mode == uint8(192) % è arrivato MAV_MODE_MANUAL_ARMED
    
    H_mav(1) = uint8(192);       % MAV_MODE_MANUAL_ARMED 
    H_mav(2) = uint8(4);         % MAV_STATE_ACTIVE
%     H_mav(3) = uint8(64);        % MAV_MODE_FLAG_MANUAL_INPUT_ENABLED
    AP_mode  = uint8([1; 0]);    % attivo il manuale  spengo l'automatico
    Base_mode_to_SF = uint8(192);
    
elseif Base_mode == uint8(208) % è arrivato MAV_MODE_STABILIZE_ARMED (sarebbe la modalità Stand By presente nello State Flow degli stati)
    
    H_mav(1) = uint8(208);       % MAV_MODE_STABILIZE_ARMED
    H_mav(2) = uint8(3);         % MAV_STATE_STANDBY
%     H_mav(3) = uint8(64);        % MAV_MODE_FLAG_MANUAL_INPUT_ENABLED
    AP_mode  = uint8([0; 0]);    % disattiva l'interruttore del manuale ma l'automatico non è ancora attivo
    Base_mode_to_SF = uint8(208);

elseif Base_mode == uint8(220) && Mav_state ~= uint8(5) % è arrivato MAV_MODE_AUTO_ARMED
    
    if (AP_int_mem(1) == uint8(0) && AP_int_mem(2) == uint8(0) && ((AP_int_mem(3) == uint8(1) || AP_int_mem(4) == uint8(1) ||...
        AP_int_mem(5) == uint8(1) || AP_int_mem(6) == uint8(1) || AP_int_mem(7) == uint8(1) || AP_int_mem(8) == uint8(1))))
    
        H_mav(1) = uint8(220);       % MAV_MODE_AUTO_ARMED
        H_mav(2) = uint8(4);         % MAV_STATE_ACTIVE
%         H_mav(3) = uint8(4);         % MAV_MODE_FLAG_AUTO_ENABLED
        AP_mode  = uint8([0; 1]);    % spengo il manuale attivo l'automatico
        Base_mode_to_SF = uint8(220);
        
    elseif (AP_int_mem(1) == uint8(0) && AP_int_mem(2) == uint8(1) && ((AP_int_mem(3) == uint8(1) || AP_int_mem(4) == uint8(1) ||...
            AP_int_mem(5) == uint8(1) || AP_int_mem(6) == uint8(1) || AP_int_mem(7) == uint8(1) || AP_int_mem(8) == uint8(1)))) 
        
        H_mav(1) = uint8(220);       % MAV_MODE_AUTO_ARMED
        H_mav(2) = uint8(4);         % MAV_STATE_ACTIVE
        AP_mode  = uint8([0; 1]);    % spengo il manuale attivo l'automatico
        Base_mode_to_SF = uint8(220);
        
    else 
        
        H_mav(1)  = uint8(208);       % MAV_MODE_STABILIZE_ARMED
        H_mav(2)  = uint8(3);         % MAV_STATE_STANDBY
        AP_mode   = uint8([0; 0]);    % attivo il manuale  spengo l'automatico
        Base_mode_to_SF = uint8(208);
    
    end

% elseif Base_mode == uint8(216)  % è arrivato MAV_MODE_GUIDED_ARMED
%     
%     H_mav(1) = uint8(8);         % MAV_MODE_FLAG_GUIDED_ENABLED
%     H_mav(2) = uint8(4);         % MAV_STATE_ACTIVE
%     AP_mode  = uint8([0; 1]);    % spengo il manuale attivo l'automatico
    
elseif Mav_state == uint8(5)  % si verifica nell'S-Function di ricezione quando il velivolo è andato in safe ovvero quando Alarm_Safe = 1
    
    H_mav(1) = uint8(220);      % MAV_MODE_AUTO_ARMED
    H_mav(2) = uint8(5);        % MAV_STATE_CRITICAL
%     H_mav(3) = uint8(128);      % MAV_MODE_FLAG_SAFETY_ARMED
    AP_mode  = uint8([0; 1]);   % spengo il manuale attivo l'automatico

% elseif Base_mode==uint8(66) % è arrivato MAV_MODE_TEST_DISARMED, lo usiamo per fare la calibrazione
%     H_mav(1)=uint8(64);        %MAV_MODE_FLAG_MANUAL_INPUT_ENABLED
%     H_mav(2)=uint8(2);         %MAV_STATE_CALIBRATING
%     AP_mode=uint8([1; 0]);     %attivo il manuale  spengo l'automatico
    
    %%%%%%%%%%%%%%%%%%%%%%%%%%%
    % elseif Base_mode==uint8(192) %%ARMED PREFLIGHT
    %     H_mav(1)=uint8(192);        %MAV_MODE_FLAG_MANUAL_INPUT_ENABLED
    %     H_mav(2)=uint8(3);          %	MAV_STATE_EMERGENCY
    %     AP_mode=uint8([0; 1]);     %spengo il manuale attivo l'automatico
    %     elseif Base_mode==uint8(64) %%DISARMED PREFLIGHT
    %     H_mav(1)=uint8(64);        %MAV_MODE_FLAG_MANUAL_INPUT_ENABLED
    %     H_mav(2)=uint8(3);          %	MAV_STATE_EMERGENCY
    %     AP_mode=uint8([0; 1]);     %spengo il manuale attivo l'automatico
    %     %%%%%%%%%%%%%%%%%%%%%%%%%%%%%%%%%%%%%%%

else
    
    H_mav(1) = uint8(192);       % MAV_MODE_MANUAL_ARMED 
    H_mav(2) = uint8(6);         % MAV_STATE_EMERGENCY
%     H_mav(3) = uint8(64);        % MAV_MODE_FLAG_MANUAL_INPUT_ENABLED
    AP_mode  = uint8([1; 0]);    % attivo il manuale  spengo l'automatico
    
end

%% parte delle informazioni sullo stato del sistema in ricezione

% calcolo dei messaggi persi provenienti dalla stazione di terra

drop_rate = 10*((100*mem_out(6))/mem_out(5));  % 10*percentuale !non moltipilicare direttamente per 10000 perchè è un uint16 e va in overflow
SyS_data  = [drop_rate mem_out(7) mem_out(3)];

%% parte per settare gli interrutori e i riferimenti

AP_int = [AP_mode; uint8(riferimenti(1:7))]; % interruttori
AP_rif = riferimenti(8:11);                  % riferimenti

T_0 = riferimenti(13); % valore della temperatura di riferimento T_0 dell'altimetro

test = test1;
